simulink model "Question1"  (R2020a)
settings: Solver=VariableStepAuto  StartTime=0.0  StopTime=10.0  RelTol=1e-3
settings Model: Creator=aishw  LastModifiedBy=aishw

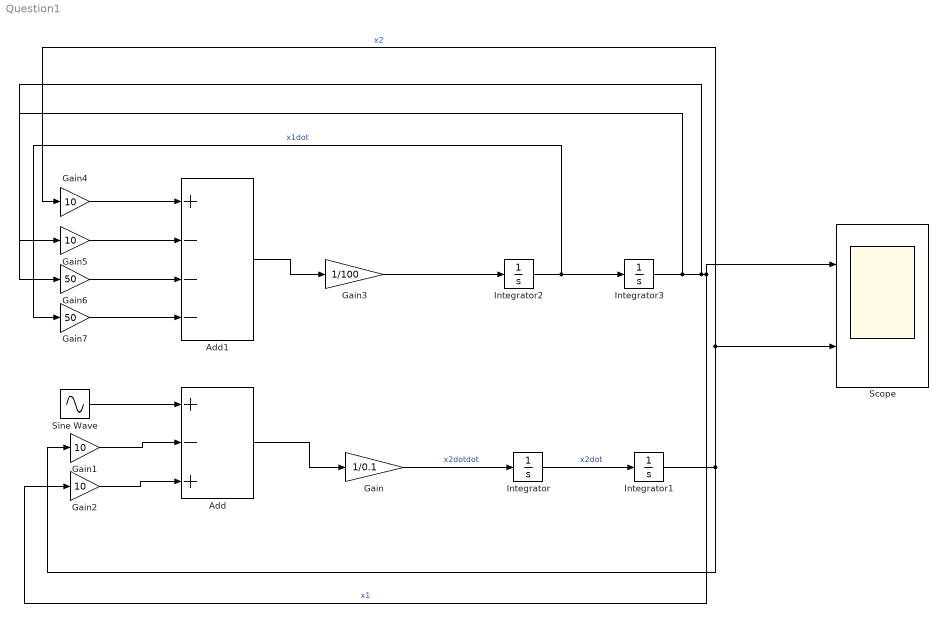
== system Question1 ==
  Add : Sum  Inputs=+-+
  Add1 : Sum  Inputs=+---
  Gain : Gain  Gain=1/0.1
  Gain{1..2,4..5} (4 alike) : Gain  Gain=10
  Gain3 : Gain  Gain=1/100
  Gain6 : Gain  Gain=50
  Gain7 : Gain  Gain=50
  Integrator{,1..3} (4 alike) : Integrator
  Scope : Scope  NumInputPorts=2
  Sine Wave : Sin  Amplitude=2  Frequency=10  SampleTime=0
  wires:
  Integrator2/1 -> Gain7/1, Integrator3/1  "x1dot"
  Integrator/1 -> Integrator1/1  "x2dot"
  Gain/1 -> Integrator/1  "x2dotdot"
  Add/1 -> Gain/1
  Integrator1/1 -> Scope/2, Gain4/1, Gain1/1  "x2"
  Integrator3/1 -> Gain6/1, Gain5/1, Gain2/1, Scope/1  "x1"
  Gain1/1 -> Add/2
  Gain2/1 -> Add/3
  Sine Wave/1 -> Add/1
  Gain3/1 -> Integrator2/1
  Add1/1 -> Gain3/1
  Gain4/1 -> Add1/1
  Gain5/1 -> Add1/2
  Gain6/1 -> Add1/3
  Gain7/1 -> Add1/4
